simulink model "f18nlclpWCsim"  (Simulink 7.2)
settings: Solver=ode45  StartTime=0.0  StopTime=10.0  RelTol=1e-3
values from neighbouring files (symbols this model uses):
  aytrim = double(subs(C(1,:)*x + D(1,:)*u,[x;u],[xtf(2:7);utf(1:3)]))    [RunF18NomSimClp.m]    (also in RunF18Sim.m = C(1,:)*xtrim(2:7) + D(1,:)*utrim(1:3))
  bdottrim = double(subs(C(end,:)*x + D(end,:)*u,[x;u],[xtf(2:7);utf(1:3)]))    [RunF18NomSimClp.m]    (also in RunF18Sim.m = C(end,:)*xtrim(2:7) + D(end,:)*utrim(1:3))
  C = Pss.C    [RunF18NomSimClp.m]    (also in RunF18Sim.m = Bank25.Pss.C)
  D = Pss.D    [RunF18NomSimClp.m]    (also in RunF18Sim.m = Bank25.Pss.D)
  d11 = ss(0)    [RunF18Sim.m]    (also in RunF18_WCsim.m = ultidyn('d11'))
  d22 = ss(0)    [RunF18Sim.m]    (also in RunF18_WCsim.m = ultidyn('d22'))
  d2r = pi/180    (= 0.0174532925199)    [f18_data.m]
  d33 = ss(0)    [RunF18Sim.m]    (also in RunF18_WCsim.m = ultidyn('d33'))
  InpPert = 0    [RunF18NomSimClp.m]    (also in RunF18Sim.m)
  K = CssR    [RunF18NomSimClp.m]    (also in RunF18Sim.m = Bank25.CssR)
  utrim = [-0.00218308158555 -0.0062308112469 -0.0468365436458 14500.0001078]    [F18Model_Coord_Phi_10.mat]    (also in F18Model_UnCoord_Phi_25.mat = [0.239553480817 0.195781713468 -0.0629449706924 14499.999992; RunF18Sim.m = Bank25.utrim)
  xtrim = [350 -3.30872252725e-24 0.272183029653 -0.00638847788994 0.00230815274318 0.0130901846893 0.174532925199 0.448024870894 0]    [F18Model_Coord_Phi_10.mat]    (also in F18Model_UnCoord_Phi_25.mat = [350 0.174532925199 0.3212281647 -0.0187468458277 0.01742146; RunF18Sim.m = Bank25.xtrim)
undefined symbols (not defined in the file or in its folder): sigbuilder_block
settings Model: Creator=chakrab  LastModifiedBy=chakrab

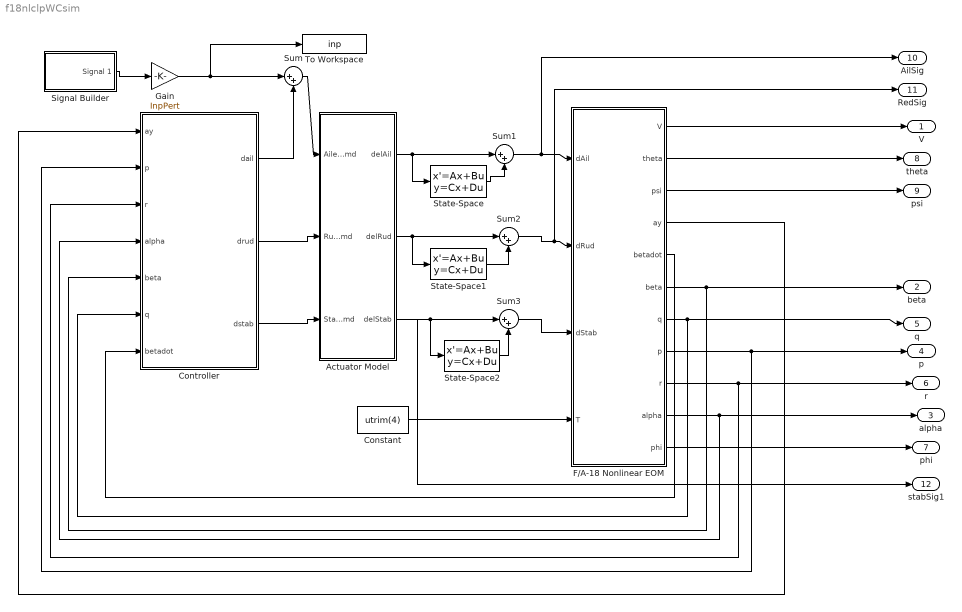
== system f18nlclpWCsim ==
  Actuator Model : Subsystem
  Constant : Constant  Value=utrim(4)  OutDataType=sfix(16)  OutScaling=2^0
  Controller : Subsystem
  F/A-18 Nonlinear EOM : Subsystem
  Gain : Gain  Gain=InpPert  ParameterDataType=sfix(16)  ParameterScaling=2^0  OutDataType=sfix(16)  OutScaling=2^0
  Signal Builder : Subsystem  Tag=STV Subsys  LoadFcn=sigbuilder_block('load');  StartFcn=sigbuilder_block('start');  StopFcn=sigbuilder_block('stop');  ClipboardFcn=sigbuilder_block('clipboard');  mask(Sigbuilder block){}
      mask help: Sigbuilder GUI
      mask init:
      | if ~strcmp(get_param(bdroot(gcbh),'SimulationStatus'),'stopped') tuvar = sigbuilder_block('maskInit'); end
      settings: CopyFcn=sigbuilder_block('copy');  DeleteFcn=sigbuilder_block('delete');  ModelCloseFcn=sigbuilder_block('modelClose');  PreSaveFcn=sigbuilder_block('preSave');  NameChangeFcn=sigbuilder_block('namechange');  OpenFcn=sigbuilder_block('open',[205.5 189.75 550.5 363.75 ]);  CloseFcn=sigbuilder_block('close');
      mask Display: plot(0,0,100,100,[10,10,40,40,10],[80,20,20,80,80],[40,10],[50,50], [40,27,10],[65,72,56],[40,25,25,10],[28,28,43,43]);
  State-Space : StateSpace  A=d11.A  B=d11.B  C=d11.C  D=d11.D
  State-Space1 : StateSpace  A=d22.a  B=d22.b  C=d22.c  D=d22.d
  State-Space2 : StateSpace  A=d33.a  B=d33.b  C=d33.c  D=d33.d
  Sum{,1..3} (4 alike) : Sum  Inputs=|++  OutDataType=sfix(16)  OutScaling=2^0
  To Workspace : ToWorkspace  VariableName=inp  SampleTime=-1  SaveFormat=Array
  V : Outport  OutDataType=sfix(16)  OutScaling=2^0
  beta : Outport  Port=2  OutDataType=sfix(16)  OutScaling=2^0
  alpha : Outport  Port=3  OutDataType=sfix(16)  OutScaling=2^0
  p : Outport  Port=4  OutDataType=sfix(16)  OutScaling=2^0
  q : Outport  Port=5  OutDataType=sfix(16)  OutScaling=2^0
  r : Outport  Port=6  OutDataType=sfix(16)  OutScaling=2^0
  phi : Outport  Port=7  OutDataType=sfix(16)  OutScaling=2^0
  theta : Outport  Port=8  OutDataType=sfix(16)  OutScaling=2^0
  psi : Outport  Port=9  OutDataType=sfix(16)  OutScaling=2^0
  AilSig : Outport  Port=10  OutDataType=sfix(16)  OutScaling=2^0
  RedSig : Outport  Port=11  OutDataType=sfix(16)  OutScaling=2^0
  stabSig1 : Outport  Port=12  OutDataType=sfix(16)  OutScaling=2^0
  wires:
  Constant/1 -> F/A-18 Nonlinear EOM/4(T)
  Actuator Model/3(delStab) -> Sum3/1, stabSig1/1, State-Space2/1
  Controller/2(drud) -> Actuator Model/2(RudderCmd)
  Controller/3(dstab) -> Actuator Model/3(StabCmd)
  F/A-18 Nonlinear EOM/8(p) -> p/1, Controller/2(p)
  F/A-18 Nonlinear EOM/9(r) -> r/1, Controller/3(r)
  F/A-18 Nonlinear EOM/10(alpha) -> alpha/1, Controller/4(alpha)
  F/A-18 Nonlinear EOM/6(beta) -> beta/1, Controller/5(beta)
  F/A-18 Nonlinear EOM/7(q) -> q/1, Controller/6(q)
  F/A-18 Nonlinear EOM/5(betadot) -> Controller/7(betadot)
  F/A-18 Nonlinear EOM/1(V) -> V/1
  F/A-18 Nonlinear EOM/2(theta) -> theta/1
  F/A-18 Nonlinear EOM/3(psi) -> psi/1
  F/A-18 Nonlinear EOM/11(phi) -> phi/1
  Signal Builder/1(Signal 1) -> Gain/1
  Controller/1(dail) -> Sum/2
  Sum/1 -> Actuator Model/1(AileronCmd)
  Gain/1 -> Sum/1, To Workspace/1
  F/A-18 Nonlinear EOM/4(ay) -> Controller/1(ay)
  Actuator Model/1(delAil) -> Sum1/1, State-Space/1
  Sum1/1 -> F/A-18 Nonlinear EOM/1(dAil), AilSig/1
  State-Space/1 -> Sum1/2
  Actuator Model/2(delRud) -> Sum2/1, State-Space1/1
  Sum2/1 -> F/A-18 Nonlinear EOM/2(dRud), RedSig/1
  State-Space1/1 -> Sum2/2
  Sum3/1 -> F/A-18 Nonlinear EOM/3(dStab)
  State-Space2/1 -> Sum3/2

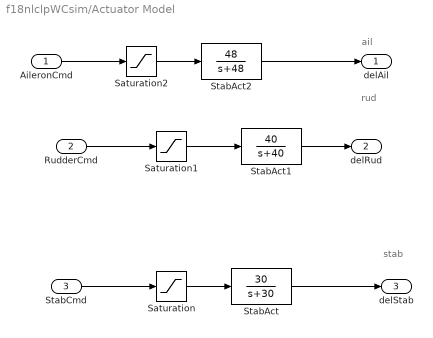
== system f18nlclpWCsim/Actuator Model ==
  note: ail
  note: rud
  note: stab
  AileronCmd : Inport
  RudderCmd : Inport  Port=2
  StabCmd : Inport  Port=3
  Saturation : Saturate  UpperLimit=10.5*d2r  LowerLimit=-24*d2r  OutDataType=sfix(16)  OutScaling=2^0
  Saturation1 : Saturate  UpperLimit=30*d2r  LowerLimit=-30*d2r  OutDataType=sfix(16)  OutScaling=2^0
  Saturation2 : Saturate  UpperLimit=45*d2r  LowerLimit=-25*d2r  OutDataType=sfix(16)  OutScaling=2^0
  StabAct : TransferFcn  Numerator=[30]  Denominator=[1 30]
  StabAct1 : TransferFcn  Numerator=[40]  Denominator=[1 40]
  StabAct2 : TransferFcn  Numerator=[48]  Denominator=[1 48]
  delAil : Outport
  delRud : Outport  Port=2
  delStab : Outport  Port=3
  wires:
  StabAct2/1 -> delAil/1
  RudderCmd/1 -> Saturation1/1
  StabCmd/1 -> Saturation/1
  Saturation/1 -> StabAct/1
  StabAct/1 -> delStab/1
  Saturation1/1 -> StabAct1/1
  StabAct1/1 -> delRud/1
  Saturation2/1 -> StabAct2/1
  AileronCmd/1 -> Saturation2/1

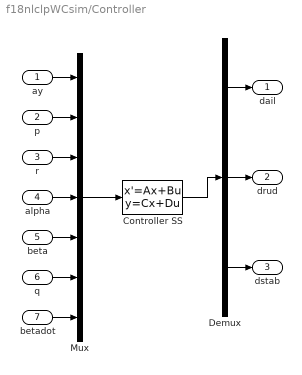
== system f18nlclpWCsim/Controller ==
  ay : Inport
  p : Inport  Port=2
  r : Inport  Port=3
  alpha : Inport  Port=4
  beta : Inport  Port=5
  q : Inport  Port=6
  betadot : Inport  Port=7
  Controller SS : StateSpace  A=K.A  B=-K.B  C=K.C  D=-K.D
  Demux : Demux  Outputs=3
  Mux : Mux  Inputs=7
  dail : Outport
  drud : Outport  Port=2
  dstab : Outport  Port=3
  wires:
  Controller SS/1 -> Demux/1
  Mux/1 -> Controller SS/1
  ay/1 -> Mux/1
  Demux/1 -> dail/1
  p/1 -> Mux/2
  r/1 -> Mux/3
  Demux/2 -> drud/1
  alpha/1 -> Mux/4
  beta/1 -> Mux/5
  Demux/3 -> dstab/1
  q/1 -> Mux/6
  betadot/1 -> Mux/7

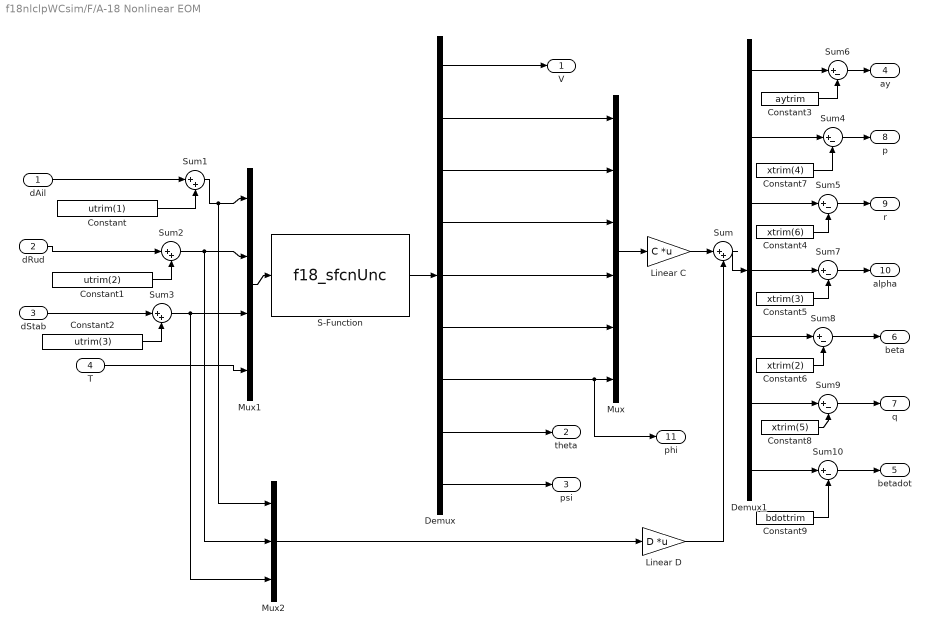
== system f18nlclpWCsim/F/A-18 Nonlinear EOM ==
  dAil : Inport
  dRud : Inport  Port=2
  dStab : Inport  Port=3
  T : Inport  Port=4
  Constant : Constant  Value=utrim(1)  OutDataType=sfix(16)  OutScaling=2^0
  Constant1 : Constant  Value=utrim(2)  OutDataType=sfix(16)  OutScaling=2^0
  Constant2 : Constant  Value=utrim(3)  OutDataType=sfix(16)  OutScaling=2^0
  Constant3 : Constant  Value=aytrim  OutDataType=sfix(16)  OutScaling=2^0
  Constant4 : Constant  Value=xtrim(6)  OutDataType=sfix(16)  OutScaling=2^0
  Constant5 : Constant  Value=xtrim(3)  OutDataType=sfix(16)  OutScaling=2^0
  Constant6 : Constant  Value=xtrim(2)  OutDataType=sfix(16)  OutScaling=2^0
  Constant7 : Constant  Value=xtrim(4)  OutDataType=sfix(16)  OutScaling=2^0
  Constant8 : Constant  Value=xtrim(5)  OutDataType=sfix(16)  OutScaling=2^0
  Constant9 : Constant  Value=bdottrim  OutDataType=sfix(16)  OutScaling=2^0
  Demux : Demux  Outputs=9
  Demux1 : Demux  Outputs=7
  Linear C : Gain  Gain=C  Multiplication=Matrix(K*u)  ParameterDataType=sfix(16)  ParameterScaling=2^0  OutDataType=sfix(16)  OutScaling=2^0
  Linear D : Gain  Gain=D  Multiplication=Matrix(K*u)  ParameterDataType=sfix(16)  ParameterScaling=2^0  OutDataType=sfix(16)  OutScaling=2^0
  Mux : Mux  Inputs=6
  Mux1 : Mux
  Mux2 : Mux  Inputs=3
  S-Function : S-Function  FunctionName=f18_sfcnUnc  Parameters=dx0 , opts  EnableBusSupport=off
  Sum{,1..3} (4 alike) : Sum  Inputs=|++  OutDataType=sfix(16)  OutScaling=2^0
  Sum{4..10} (7 alike) : Sum  Inputs=|+-  OutDataType=sfix(16)  OutScaling=2^0
  V : Outport
  theta : Outport  Port=2
  psi : Outport  Port=3
  ay : Outport  Port=4  OutDataType=sfix(16)  OutScaling=2^0
  betadot : Outport  Port=5  OutDataType=sfix(16)  OutScaling=2^0
  beta : Outport  Port=6
  q : Outport  Port=7
  p : Outport  Port=8
  r : Outport  Port=9
  alpha : Outport  Port=10
  phi : Outport  Port=11
  wires:
  Mux1/1 -> S-Function/1
  S-Function/1 -> Demux/1
  Demux/1 -> V/1
  Demux/5 -> Mux/4
  Demux/2 -> Mux/1
  Demux/3 -> Mux/2
  Demux/4 -> Mux/3
  Demux/6 -> Mux/5
  T/1 -> Mux1/4
  Demux/7 -> Mux/6, phi/1
  Demux/8 -> theta/1
  Demux/9 -> psi/1
  Mux/1 -> Linear C/1
  Mux2/1 -> Linear D/1
  Linear C/1 -> Sum/1
  Linear D/1 -> Sum/2
  Sum/1 -> Demux1/1
  dAil/1 -> Sum1/1
  Sum1/1 -> Mux1/1, Mux2/1
  dRud/1 -> Sum2/1
  Sum2/1 -> Mux1/2, Mux2/2
  dStab/1 -> Sum3/1
  Sum3/1 -> Mux1/3, Mux2/3
  Constant/1 -> Sum1/2
  Constant1/1 -> Sum2/2
  Constant2/1 -> Sum3/2
  Demux1/1 -> Sum6/1
  Sum6/1 -> ay/1
  Constant3/1 -> Sum6/2
  Demux1/2 -> Sum4/1
  Sum4/1 -> p/1
  Sum5/1 -> r/1
  Demux1/3 -> Sum5/1
  Sum7/1 -> alpha/1
  Demux1/4 -> Sum7/1
  Sum8/1 -> beta/1
  Demux1/5 -> Sum8/1
  Demux1/6 -> Sum9/1
  Sum9/1 -> q/1
  Demux1/7 -> Sum10/1
  Sum10/1 -> betadot/1
  Constant7/1 -> Sum4/2
  Constant4/1 -> Sum5/2
  Constant5/1 -> Sum7/2
  Constant6/1 -> Sum8/2
  Constant8/1 -> Sum9/2
  Constant9/1 -> Sum10/2

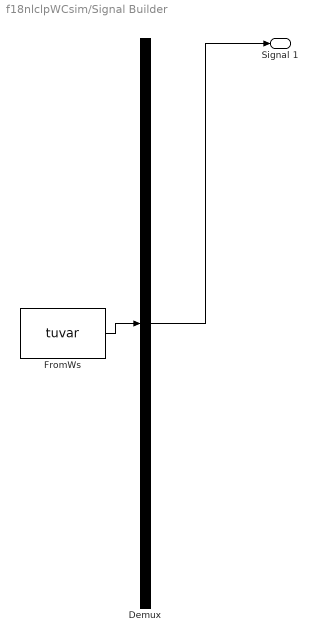
== system f18nlclpWCsim/Signal Builder ==
  Demux : Demux  Tag=STV Demux  Outputs=1
  FromWs : FromWorkspace  Tag=STV FromWs  VariableName=tuvar  SampleTime=0  SigBuilderData=DataTag0  VnvData=DataTag1
      SigBuilderData=|
      | common.afterFinalStr = 'Extrapolate'
      | common.sampleTime = 0
      | dataSet.timeRange = [0 10]
      | dataSet.name = 'Group 1'
      | sbobj.Groups.Signals.XData = [0 1 1 2 2 3 3 10]
      | sbobj.Groups.Signals.YData = [0 0 0.1 0.1 -0.1 -0.1 0 0]
  Signal 1 : Outport  Tag=STV Outport  OutDataType=sfix(16)  OutScaling=2^0
  wires:
  Demux/1 -> Signal 1/1
  FromWs/1 -> Demux/1
